simulink model "Pump_test"  (R2014b)
settings: Solver=ode23tb  StartTime=0.0  StopTime=100  RelTol=1e-3
libraries: DAEMOT_Lib x3
settings Model: Creator=pangbor2  LastModifiedBy=koeln2

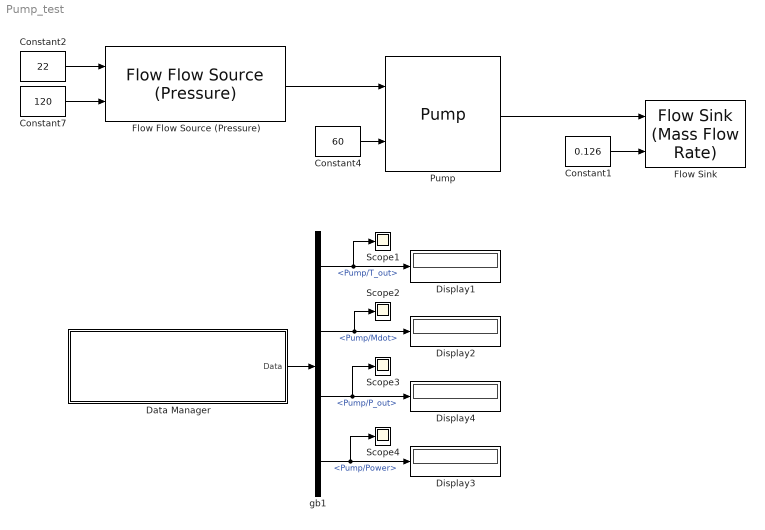
== system Pump_test ==
  Constant1 : Constant  Value=0.126
  Constant2 : Constant  Value=22
  Constant4 : Constant  Value=60
  Constant7 : Constant  Value=120
  Data Manager : Subsystem  AncestorBlock=DAEMOT_Lib/Support Functions/Data Manager  mask{null=0}
      mask init:
      | set_param(gcb, 'LinkStatus', 'inactive')    % disable the library link
      settings: OpenFcn=data_manager
      mask Display: str ='Pump/T_out\nPump/Mdot\nPump/P_out\nPump/Power'; fprintf(str)
  Display{1..4} (4 alike) : Display
  Flow Flow Source (Pressure) : DAEMOT_Lib/Components/Flow Flow Source (Pressure)  M_ext=on  M=0  T_ext=on  T=0  P_ext=on  P=0
  Flow Sink : DAEMOT_Lib/Components/Flow Sink (Mass Flow Rate)  M_ext=on  M=0  T_ext=on  T=0  P_ext=on  P=0
  Pump : DAEMOT_Lib/Components/Pump  fld=PG50  pump=PumpProp.mat  P_init=145  T_init=22  H=0  D=13*1e-3  L=0.1  t=0.0015  E=2.4e6  v=5e-6
  Scope{1..4} (4 alike) : Scope
      Scope3 settings: SaveName=ScopeData2
      Scope4 settings: SaveName=ScopeData3
  gb1 : BusSelector  OutputSignals=Pump/T_out,Pump/Mdot,Pump/P_out,Pump/Power
  wires:
  Constant4/1 -> Pump/2
  Data Manager/1(Data) -> gb1/1
  gb1/1 -> Scope1/1, Display1/1  "<Pump/T_out>"
  gb1/2 -> Scope2/1, Display2/1  "<Pump/Mdot>"
  gb1/4 -> Scope4/1, Display3/1  "<Pump/Power>"
  Flow Flow Source (Pressure)/1 -> Pump/1
  Constant7/1 -> Flow Flow Source (Pressure)/2
  Constant2/1 -> Flow Flow Source (Pressure)/1
  Constant1/1 -> Flow Sink/2
  Pump/1 -> Flow Sink/1
  gb1/3 -> Scope3/1, Display4/1  "<Pump/P_out>"

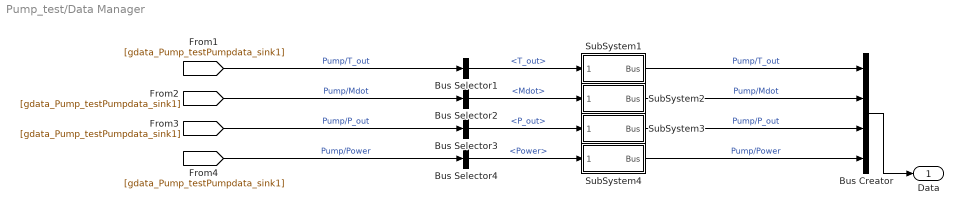
== system Pump_test/Data Manager ==
  Bus Creator : BusCreator
  Bus Selector1 : BusSelector  OutputSignals=T_out
  Bus Selector2 : BusSelector  OutputSignals=Mdot
  Bus Selector3 : BusSelector  OutputSignals=P_out
  Bus Selector4 : BusSelector  OutputSignals=Power
  SubSystem1 : Subsystem
  SubSystem2 : Subsystem
  SubSystem3 : Subsystem
  SubSystem4 : Subsystem
  Data : Outport
  wires:
  Bus Creator/1 -> Data/1
  [gdata_Pump_testPumpdata_sink1] -> Bus Selector1/1  "Pump/T_out"
  Bus Selector1/1 -> SubSystem1/1(Rename)  "<T_out>"
  SubSystem1/1(Bus) -> Bus Creator/1  "Pump/T_out"
  [gdata_Pump_testPumpdata_sink1] -> Bus Selector2/1  "Pump/Mdot"
  Bus Selector2/1 -> SubSystem2/1(Rename)  "<Mdot>"
  SubSystem2/1(Bus) -> Bus Creator/2  "Pump/Mdot"
  [gdata_Pump_testPumpdata_sink1] -> Bus Selector3/1  "Pump/P_out"
  Bus Selector3/1 -> SubSystem3/1(Rename)  "<P_out>"
  SubSystem3/1(Bus) -> Bus Creator/3  "Pump/P_out"
  [gdata_Pump_testPumpdata_sink1] -> Bus Selector4/1  "Pump/Power"
  Bus Selector4/1 -> SubSystem4/1(Rename)  "<Power>"
  SubSystem4/1(Bus) -> Bus Creator/4  "Pump/Power"

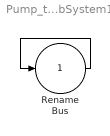
== system Pump_test/Data Manager/SubSystem1 ==
  Rename : Inport
  Bus : Outport
  wires:
  Rename/1 -> Bus/1

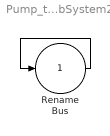
== system Pump_test/Data Manager/SubSystem2 ==
  Rename : Inport
  Bus : Outport
  wires:
  Rename/1 -> Bus/1

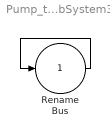
== system Pump_test/Data Manager/SubSystem3 ==
  Rename : Inport
  Bus : Outport
  wires:
  Rename/1 -> Bus/1

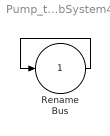
== system Pump_test/Data Manager/SubSystem4 ==
  Rename : Inport
  Bus : Outport
  wires:
  Rename/1 -> Bus/1
